simulink model "NoTrailer"  (R2026b)
settings: Solver=VariableStepAuto
settings Model: ModifiedByFormat=The MathWorks, Inc.  Creator=The MathWorks, Inc.  LastModifiedBy=The MathWorks, Inc.

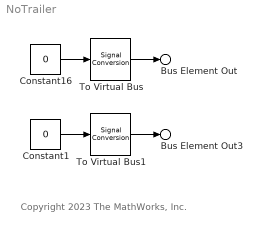
== system NoTrailer ==
  note: Copyright 2023 The MathWorks, Inc.
  Constant1 : Constant  Value=0  OutDataTypeStr=Bus: TrlrWheelsBUS  SampleTime=Inf
  Constant16 : Constant  Value=0  OutDataTypeStr=Bus: TrlrBodyBUS  SampleTime=Inf
  To Virtual Bus : SignalConversion  ConversionOutput=Virtual bus  OverrideOpt=off
  To Virtual Bus1 : SignalConversion  ConversionOutput=Virtual bus  OverrideOpt=off
  Bus Element Out3 : Outport  PortName=Wheels
  Bus Element Out : Outport  Port=2  PortName=TrlrBody
  wires:
  To Virtual Bus1/1 -> Bus Element Out3/1
  To Virtual Bus/1 -> Bus Element Out/1
  Constant1/1 -> To Virtual Bus1/1
  Constant16/1 -> To Virtual Bus/1
